simulink model "moving_average"  (R2023b)
settings: Solver=VariableStepAuto  StartTime=0.0  StopTime=10.0  RelTol=1e-3
values from neighbouring files (symbols this model uses):
  M = 5    [Lab1_Es1.m]
  Ts = 0.1    [Lab1_Es1.m]
settings Model: Creator=alberto  LastModifiedBy=alberto

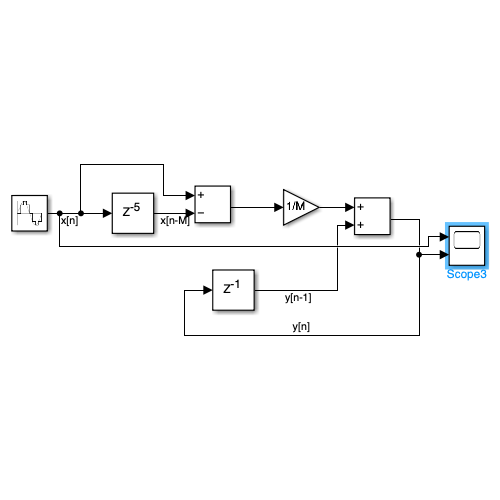
[thumbnail: Simulink's stored preview of the top-level diagram]
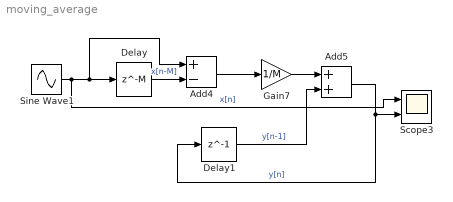
== system moving_average ==
  Add4 : Sum  Inputs=+-
  Add5 : Sum
  Delay : Delay  DelayLength=M
  Delay1 : Delay  DelayLength=1
  Gain7 : Gain  Gain=1/M
  Scope3 : Scope  NumInputPorts=2
  Sine Wave1 : Sin  Frequency=2*pi  SampleTime=Ts
  wires:
  Add4/1 -> Gain7/1
  Delay/1 -> Add4/2  "x[n-M]"
  Add5/1 -> Scope3/2, Delay1/1  "y[n]"
  Sine Wave1/1 -> Scope3/1, Add4/1, Delay/1  "x[n]"
  Gain7/1 -> Add5/1
  Delay1/1 -> Add5/2  "y[n-1]"
